simulink model "TestingModel"  (R2022a)
settings: Solver=VariableStepAuto  StartTime=0.0  StopTime=10.0  RelTol=1e-3
settings Model: Creator=LEGION  LastModifiedBy=LEGION

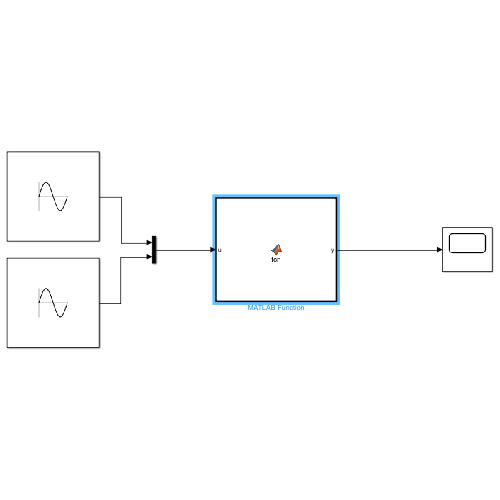
[thumbnail: Simulink's stored preview of the top-level diagram]
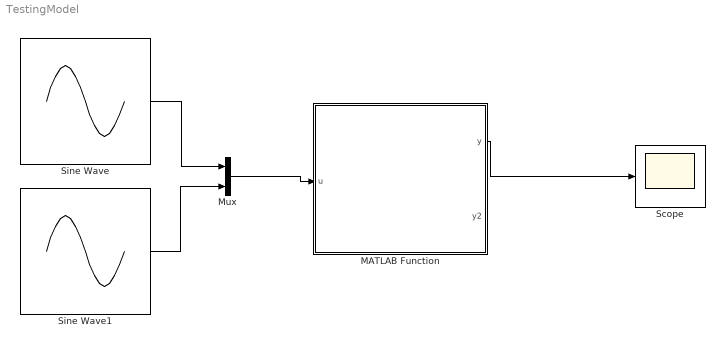
== system TestingModel ==
  MATLAB Function : MATLAB Function  TreatAsAtomicUnit=on
  Mux : Mux  Inputs=2
  Scope : Scope
  Sine Wave : Sin  SampleTime=0
  Sine Wave1 : Sin  Amplitude=2  Frequency=0.5  SampleTime=0
  wires:
  Sine Wave/1 -> Mux/1
  MATLAB Function/1(y) -> Scope/1
  Sine Wave1/1 -> Mux/2
  Mux/1 -> MATLAB Function/1(u)

== matlab function TestingModel/MATLAB Function ==
  data: u input; y output; y2 output
function [y, y2] = fcn(u)

n_data = 2;
y = u(n_data);
y2 = u(1);
